simulink model "dbuildv3p1"  (R2024b)
settings: Solver=FixedStepAuto  StartTime=0.0  StopTime=inf  FixedStep=0.001  RelTol=1e-3
model workspace (MAT data in the model file):
  A_busbar = 0.0015
  A_pack = 0.711626248
  C = 400
  C_nominal = 3
  GR = 13.75
  I_max = 157.708978328
  Izz = 76.97
  M = 251.54
  P = 5
  P_DD = 1
  REGEN_GAIN = 0
  R_e = 0.197
  S = 138
  SW_TV_GAIN = 0.0250298750679
  SoC_initial = 1
  TC_CUT = 500
  T_amb = 296.15
  Tmax = 21
  W = 1.53
  W_max = 34
  a = 0.7497
  brakebias = 0.5
  busbar_CC_area = 0.000108
  busbar_Cp = 237
  busbar_length = 0.032
  busbar_mass = 0.01
  busbar_resistivity = 1.68e-08
  busbar_thermalcontact_resistance = 1
  c_factor = 0.244
  cell_Cp = 1000
  cell_mass = 0.046
  deg_to_rad = 0.0174533
  g = 9.81
  h = 0.253
  h_busbar = 5
  h_pack = 5
  kappa_thresh = 0.09
  l = 1.53
  mpersec_to_kph = 3.6
  rackdisp_to_steerangle = 1.29615626969
  rad_to_deg = 57.2958
  rpm_to_radpers = 0.10472
  t = 1.2
  trigger_pressure = 4.65396
undefined symbols (not defined in the file or in its folder): TC_switch, TV_switch
libraries: eeGeneralControl x2, Solver_SF x1, sl3dlib x1, simulink x1
(part 2 of 2)

== system dbuildv3p1/Control System/Driver Assists/Traction Control/Slip Ratio Calculator/Wheel Center Speed Calculator ==
  Gain : Gain  Gain=t/2
  Gain1 : Gain  Gain=deg_to_rad
  Mux : Mux  Inputs=2
  Sum : Sum  Inputs=|++
  Sum1 : Sum  Inputs=|+-
  Calculated Wheel Center Velocity (m/s) : Outport
  wires:
  [r] -> Gain1/1  "Yaw Rate (deg/s)"
  [Vx] -> Sum1/1, Sum/2  "Vehicle Velocity (m/s)"
  Mux/1 -> Calculated Wheel Center Velocity (m/s)/1
  Gain/1 -> Sum/1, Sum1/2
  Sum1/1 -> Mux/1  "RL WC Velocity (m/s)"
  Gain1/1 -> Gain/1  "Yaw Rate (rad/s)"
  Sum/1 -> Mux/2  "RR WC Velocity (m/s)"

== system dbuildv3p1/Control System/Driver Assists/Traction Control/Tire Load Calculator/Lateral Load Transfer ==
  Constant : Constant  Value=h
  Constant1 : Constant  Value=t
  Divide : Product  Inputs=*/
  Gain1 : Gain  Gain=M*g*(a/l)
  Gain2 : Gain  Gain=M*g*(1- (a/l))
  Product : Product
  Front Lateral Load Transfer (N) : Outport
  Rear Lateral Load Transfer (N) : Outport  Port=2
  wires:
  [Ay] -> Product/1  "Lateral Acceleration (G)"
  Constant/1 -> Product/2  "CG Height (m)"
  Product/1 -> Divide/1
  Constant1/1 -> Divide/2  "Trackwidth (m)"
  Gain1/1 -> Front Lateral Load Transfer (N)/1  "Front Lateral Load Transfer (N)"
  Divide/1 -> Gain2/1, Gain1/1
  Gain2/1 -> Rear Lateral Load Transfer (N)/1  "Rear Lateral Load Transfer (N)"

== system dbuildv3p1/Control System/Driver Assists/Traction Control/Tire Load Calculator/Longitudinal Load Transfer ==
  Gain : Gain  Gain=-h/W
  Gain1 : Gain  Gain=M*g
  Longitudinal Load Transfer (N) : Outport
  wires:
  [Ax] -> Gain/1
  Gain/1 -> Gain1/1
  Gain1/1 -> Longitudinal Load Transfer (N)/1

== system dbuildv3p1/Control System/Driver Assists/Traction Control/Vx Estimation/Ax to Vx ==
  Ax : Inport
  Omega Vx : Inport  Port=2
  Enable : EnablePort
  Integrator : Integrator
  Plus : Sum
  to m/s^2 : Gain  Gain=g
  Ax Vx : Outport
  wires:
  Ax/1 -> to m/s^2/1
  Integrator/1 -> Plus/2
  Omega Vx/1 -> Plus/1
  Plus/1 -> Ax Vx/1
  to m/s^2/1 -> Integrator/1

== system dbuildv3p1/Control System/Driver Assists/Traction Control/Vx Estimation/Method Enabler ==
  BRK_F : Inport
  Constant : Constant  Value=0
  Constant1 : Constant
  Constant2 : Constant  Value=0
  Constant3 : Constant
  Switch : Switch  Criteria=u2 > Threshold  Threshold=0.1  SaturateOnIntegerOverflow=off  InputSameDT=off
  Switch1 : Switch  Criteria=u2 > Threshold  SaturateOnIntegerOverflow=off  InputSameDT=off
  Enable Ax method : Outport
  Enable omega method : Outport  Port=2
  wires:
  Constant1/1 -> Switch/3
  Constant/1 -> Switch/1
  BRK_F/1 -> Switch/2
  Constant2/1 -> Switch1/1
  Constant3/1 -> Switch1/3
  Switch1/1 -> Enable Ax method/1
  Switch/1 -> Enable omega method/1, Switch1/2

== system dbuildv3p1/Control System/Driver Assists/Traction Control/Vx Estimation/omega to Vx ==
  omega : Inport
  Front Axle Circumference : Inport  Port=2
  Enable : EnablePort
  Gain1 : Gain  Gain=1/60
  Product : Product
  Vx : Outport
  wires:
  omega/1 -> Gain1/1
  Product/1 -> Vx/1
  Gain1/1 -> Product/1
  Front Axle Circumference/1 -> Product/2

== system dbuildv3p1/DiL Functionality/Driver inputs/Button Box/TC control/If Action Subsystem ==
  Action Port : ActionPort
  Add : Sum
  Constant1 : Constant  Value=-1
  Constant2 : Constant
  Display : Display
  Memory : Memory  InitialCondition=TC_switch  LinearizeMemory=on
  Switch : Switch  Criteria=u2 > Threshold  SaturateOnIntegerOverflow=off  InputSameDT=off
  TC switch : Outport
  wires:
  Constant2/1 -> Switch/3
  Constant1/1 -> Switch/1
  Memory/1 -> TC switch/1, Display/1, Switch/2, Add/1
  Add/1 -> Memory/1
  Switch/1 -> Add/2

== system dbuildv3p1/DiL Functionality/Driver inputs/Button Box/TV control/If Action Subsystem ==
  Action Port : ActionPort
  Add : Sum
  Constant1 : Constant  Value=-1
  Constant2 : Constant
  Display : Display
  Memory : Memory  InitialCondition=TV_switch  LinearizeMemory=on
  Switch : Switch  Criteria=u2 > Threshold  SaturateOnIntegerOverflow=off  InputSameDT=off
  TV switch : Outport
  wires:
  Constant2/1 -> Switch/3
  Constant1/1 -> Switch/1
  Memory/1 -> TV switch/1, Display/1, Switch/2, Add/1
  Add/1 -> Memory/1
  Switch/1 -> Add/2

== system dbuildv3p1/Battery Thermal Model/Battery Cells/Battery Heat Generation/Pack Current/Sony VTC6 Equivalent Circuit/Equivalent Circuit Look Ups ==
  Pack SoC (-) : Inport
  Cell C-Rate (-) : Inport  Port=2
  C1 LUT : Lookup_n-D  BreakpointsForDimension1=[0.1;0.2;0.3;0.4;0.5;0.6;0.7;0.8;0.9;1]  BreakpointsForDimension2=[-10;-5;-1;-0.333;0.333;1;2;3]  Table=[0.018906 0.021356 0.02305 0.022911 0.023301 0.023001 0.022654 0.019898;0.01868 0.020344 0.020909 0.020815 0.020944 0.020599 0.020712 0.017891;0.018453 0.019332 0.018859 0.023564 0.020028 0.019683 0.018901 0.017366;0.018226 0.019017 0.019644 0.020423 0.019635 0.019161 0.018682 0.01725;0.017999 0.018694 0.019687 0.020161 0.019897 0.01894 0.018442 0.01725;0.017916 0.018598 0.018989 0.01859 0.019505 0.018506 0.018289 0.017251;0.017743 0.018319 0.018291 0.022256 0.019767 0.018636 0.017788 0.017251;0.018183 0.018773 0.019295 0.021996 0.019898 0.019336 0.017286 0.017251;0.019549 0.020642 0.021608 0.025136 0.022253 0.020993 0.016785 0.017251;0.022703 0.024917 0.026536 0.026706 0.024609 0.02265 0.016283 0.017251]  ExtrapMethod=Clip  InternalRulePriority=Speed  RndMeth=Simplest
      settings: InputPortMap=u0,u1
  OCV : Lookup_n-D  NumberOfTableDimensions=1  BreakpointsForDimension1=[0.1;0.2;0.3;0.4;0.5;0.6;0.7;0.8;0.9;1]  BeginIndexSearchUsingPreviousIndexResult=on  Table=[3.227877;3.437376;3.537935;3.663634;3.755814;3.835423;3.940172;4.047017;4.097296;4.187904]  InternalRulePriority=Speed  RndMeth=Simplest
  R0 LUT : Lookup_n-D  BreakpointsForDimension1=[0.1;0.2;0.3;0.4;0.5;0.6;0.7;0.8;0.9;1]  BreakpointsForDimension2=[-10;-5;-1;-0.333;0.333;1;2;3]  Table=[0.018906 0.021356 0.02305 0.022911 0.023301 0.023001 0.022654 0.019898;0.01868 0.020344 0.020909 0.020815 0.020944 0.020599 0.020712 0.017891;0.018453 0.019332 0.018859 0.023564 0.020028 0.019683 0.018901 0.017366;0.018226 0.019017 0.019644 0.020423 0.019635 0.019161 0.018682 0.01725;0.017999 0.018694 0.019687 0.020161 0.019897 0.01894 0.018442 0.01725;0.017916 0.018598 0.018989 0.01859 0.019505 0.018506 0.018289 0.017251;0.017743 0.018319 0.018291 0.022256 0.019767 0.018636 0.017788 0.017251;0.018183 0.018773 0.019295 0.021996 0.019898 0.019336 0.017286 0.017251;0.019549 0.020642 0.021608 0.025136 0.022253 0.020993 0.016785 0.017251;0.022703 0.024917 0.026536 0.026706 0.024609 0.02265 0.016283 0.017251]  ExtrapMethod=Clip  InternalRulePriority=Speed  RndMeth=Simplest
      settings: InputPortMap=u0,u1
  R1 LUT : Lookup_n-D  BreakpointsForDimension1=[0.1;0.2;0.3;0.4;0.5;0.6;0.7;0.8;0.9;1]  BreakpointsForDimension2=[-10;-5;-1;-0.333;0.333;1;2;3]  Table=[0.018906 0.021356 0.02305 0.022911 0.023301 0.023001 0.022654 0.019898;0.01868 0.020344 0.020909 0.020815 0.020944 0.020599 0.020712 0.017891;0.018453 0.019332 0.018859 0.023564 0.020028 0.019683 0.018901 0.017366;0.018226 0.019017 0.019644 0.020423 0.019635 0.019161 0.018682 0.01725;0.017999 0.018694 0.019687 0.020161 0.019897 0.01894 0.018442 0.01725;0.017916 0.018598 0.018989 0.01859 0.019505 0.018506 0.018289 0.017251;0.017743 0.018319 0.018291 0.022256 0.019767 0.018636 0.017788 0.017251;0.018183 0.018773 0.019295 0.021996 0.019898 0.019336 0.017286 0.017251;0.019549 0.020642 0.021608 0.025136 0.022253 0.020993 0.016785 0.017251;0.022703 0.024917 0.026536 0.026706 0.024609 0.02265 0.016283 0.017251]  InternalRulePriority=Speed  RndMeth=Simplest
      settings: InputPortMap=u0,u1
  Terminator : Terminator
  Terminator1 : Terminator
  OCV (V) : Outport
  R0 Resistance (ohms) : Outport  Port=2
  wires:
  Cell C-Rate (-)/1 -> R1 LUT/2, R0 LUT/2, C1 LUT/2
  Pack SoC (-)/1 -> OCV/1, C1 LUT/1, R1 LUT/1, R0 LUT/1
  C1 LUT/1 -> Terminator/1  "C1 Capacitance (farads)"
  R1 LUT/1 -> Terminator1/1  "R1 Resistance (ohms)"
  R0 LUT/1 -> R0 Resistance (ohms)/1  "R0 Resistance (ohms)"
  OCV/1 -> OCV (V)/1

== system dbuildv3p1/Control System/Driver Assists/Torque Vectoring/Target Yaw Rate Estimator/Slip Angle Estimator/Front ==
  Atan : Trigonometry  Operator=atan
  Constant : Constant  Value=a
  Divide : Product  Inputs=*/
  Divide1 : Product  Inputs=*/
  Gain : Gain  Gain=c_factor
  Gain1 : Gain  Gain=rackdisp_to_steerangle
  Gain2 : Gain  Gain=1/3.6
  Gain3 : Gain  Gain=g
  Square : Math  Operator=square
  Sum : Sum  Inputs=|+-
  tag scope: alpha_F=global
  wires:
  [delta_SW] -> Gain/1  "Steering Wheel Angle (deg)"
  Gain/1 -> Gain1/1  "Rack Displacement (mm)"
  Gain1/1 -> Sum/2  "Front Wheel Steering Angle (deg)"
  [Vx] -> Gain2/1  "Vehicle Velocity (kph)"
  Gain2/1 -> Square/1  "Vehicle Velocity (m/s)"
  Square/1 -> Divide/1
  [Ay] -> Gain3/1  "Lateral Acceleration (G)"
  Gain3/1 -> Divide/2  "Lateral Acceleration (m/s^2)"
  Divide/1 -> Divide1/2  "Turning Radius (m)"
  Constant/1 -> Divide1/1  "CG to Front Wheel Distance (m)"
  Atan/1 -> Sum/1  "Slip Angle w/o Steering (deg)"
  Divide1/1 -> Atan/1
  Sum/1 -> [alpha_F]  "Front Wheel Slip Angle (deg)"

== system dbuildv3p1/Control System/Driver Assists/Torque Vectoring/Target Yaw Rate Estimator/Slip Angle Estimator/Rear ==
  Atan : Trigonometry  Operator=atan
  Constant : Constant  Value=l-a
  Divide : Product  Inputs=*/
  Divide1 : Product  Inputs=*/
  Gain2 : Gain  Gain=1/3.6
  Gain3 : Gain  Gain=g
  Square : Math  Operator=square
  tag scope: alpha_R=global
  wires:
  Divide/1 -> Divide1/2  "Turning Radius (m)"
  [Ay] -> Gain3/1  "Lateral Acceleration (G)"
  Atan/1 -> [alpha_R]  "Rear Wheel Slip Angle (deg)"
  Gain3/1 -> Divide/2  "Lateral Acceleration (m/s^2)"
  [Vx] -> Gain2/1  "Vehicle Velocity (kph)"
  Square/1 -> Divide/1
  Constant/1 -> Divide1/1  "CG to Rear Wheel Distance (m)"
  Gain2/1 -> Square/1  "Vehicle Velocity (m/s)"
  Divide1/1 -> Atan/1
